simulink model "INCREMENTAL_ENCODER"  (R2019b)
settings: Solver=VariableStepAuto  StartTime=0.0  StopTime=10.0  RelTol=1e-3
undefined symbols (not defined in the file): Ne
libraries: simulink_extras x5, simulink x2
settings Model: Creator=simone  LastModifiedBy=simone
settings ModelReferenceCC: ModelReferenceNumInstancesAllowed=Single

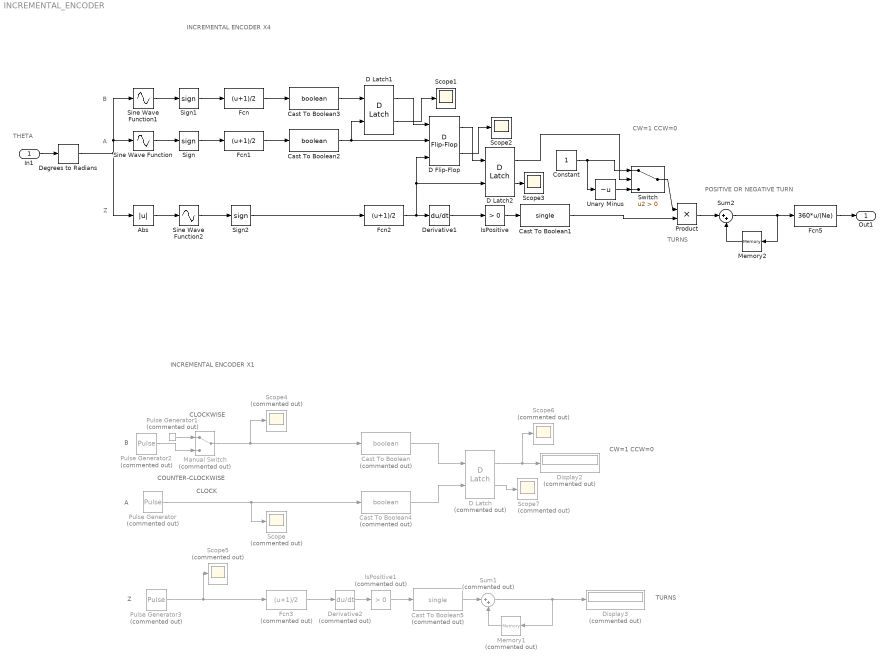
== system INCREMENTAL_ENCODER ==
  note: POSITIVE OR NEGATIVE TURN
  note: THETA
  note: Z
  note: B
  note: CW=1
      | CCW=0
  note: A
  note: INCREMENTAL ENCODER X4
  note: B
  note: TURNS
  note: Z
  note: COUNTER-CLOCKWISE
  note: A
  note: CLOCK
  note: CLOCKWISE
  note: CW=1
      |
      | CCW=0
  note: INCREMENTAL ENCODER X1
  note: TURNS
  In1 : Inport
  Abs : Abs
  Cast To Boolean : DataTypeConversion  Commented=on  OutDataTypeStr=boolean
  Cast To Boolean1 : DataTypeConversion  OutDataTypeStr=single  RndMeth=Zero
  Cast To Boolean2 : DataTypeConversion  OutDataTypeStr=boolean
  Cast To Boolean3 : DataTypeConversion  OutDataTypeStr=boolean  RndMeth=Zero
  Cast To Boolean4 : DataTypeConversion  Commented=on  OutDataTypeStr=boolean
  Cast To Boolean5 : DataTypeConversion  Commented=on  OutDataTypeStr=single  RndMeth=Zero
  Constant : Constant
  D Flip-Flop : simulink_extras/Flip Flops/D Flip-Flop
      settings: SourceProductName=Simulink
  D Latch : simulink_extras/Flip Flops/D Latch  Commented=on
      settings: SourceProductName=Simulink  SourceProductBaseCode=SL
  D Latch1 : simulink_extras/Flip Flops/D Latch
      settings: SourceProductName=Simulink  SourceProductBaseCode=SL
  D Latch2 : simulink_extras/Flip Flops/D Latch
      settings: SourceProductName=Simulink  SourceProductBaseCode=SL
  Degrees to Radians : simulink_extras/Transformations/Degrees to Radians
  Derivative1 : Derivative
  Derivative2 : Derivative  Commented=on
  Display2 : Display  Commented=on
  Display3 : Display  Commented=on
  Fcn : Fcn  Expr=(u+1)/2
  Fcn1 : Fcn  Expr=(u+1)/2
  Fcn2 : Fcn  Expr=(u+1)/2
  Fcn3 : Fcn  Commented=on  Expr=(u+1)/2
  Fcn5 : Fcn  Expr=360*u/(Ne)
  IsPositive : simulink/Logic and Bit Operations/Compare To Zero  relop=>  OutDataTypeStr=boolean
  IsPositive1 : simulink/Logic and Bit Operations/Compare To Zero  Commented=on  relop=>  OutDataTypeStr=boolean
  Manual Switch : ManualSwitch  Commented=on
  Memory1 : Memory  Commented=on  InheritSampleTime=on  LinearizeMemory=on  LinearizeAsDelay=on
  Memory2 : Memory  InitialCondition=-1  InheritSampleTime=on  LinearizeMemory=on  LinearizeAsDelay=on
  Product : Product
  Pulse Generator : DiscretePulseGenerator  Commented=on  PulseType=Time based  Period=1  PulseWidth=50
  Pulse Generator1 : DiscretePulseGenerator  Commented=on  PulseType=Time based  Period=1  PulseWidth=50  PhaseDelay=-0.25
  Pulse Generator2 : DiscretePulseGenerator  Commented=on  PulseType=Time based  Period=1  PulseWidth=50  PhaseDelay=0.25
  Pulse Generator3 : DiscretePulseGenerator  Commented=on  PulseType=Time based  PhaseDelay=2
  Scope{,4..7} (5 alike) : Scope  Commented=on
  Scope1 : Scope
  Scope2 : Scope
  Scope3 : Scope
  Sign : Signum
  Sign1 : Signum
  Sign2 : Signum
  Sine Wave Function : Sin  TimeSource=Use external signal  Frequency=Ne  SampleTime=0
  Sine Wave Function1 : Sin  TimeSource=Use external signal  Frequency=Ne  Phase=-pi/2  SampleTime=0
  Sine Wave Function2 : Sin  TimeSource=Use external signal  Frequency=Ne  SampleTime=0
  Sum1 : Sum  Commented=on  Inputs=|++
  Sum2 : Sum  Inputs=|++
  Switch : Switch  Criteria=u2 > Threshold
  Unary Minus : UnaryMinus
  Out1 : Outport
  wires:
  Degrees to Radians/1 -> Sine Wave Function1/1, Sine Wave Function/1, Abs/1
  Cast To Boolean2/1 -> D Latch1/2, D Flip-Flop/2
  Sign/1 -> Fcn1/1
  Fcn/1 -> Cast To Boolean3/1
  Sign1/1 -> Fcn/1
  D Flip-Flop/1 -> D Latch2/1
  Fcn1/1 -> Cast To Boolean2/1
  Sign2/1 -> Fcn2/1
  IsPositive/1 -> Cast To Boolean1/1
  Sine Wave Function1/1 -> Sign1/1
  Sum2/1 -> Memory2/1, Fcn5/1
  Memory2/1 -> Sum2/2
  Abs/1 -> Sine Wave Function2/1
  Sine Wave Function2/1 -> Sign2/1
  Derivative1/1 -> IsPositive/1
  Fcn2/1 -> D Flip-Flop/3, D Latch2/2, Derivative1/1
  Sine Wave Function/1 -> Sign/1
  In1/1 -> Degrees to Radians/1
  D Latch1/1 -> D Flip-Flop/1
  Cast To Boolean3/1 -> D Latch1/1
  Pulse Generator3/1 -> Scope5/1, Fcn3/1
  Cast To Boolean5/1 -> Sum1/1
  Sum1/1 -> Memory1/1, Display3/1
  Derivative2/1 -> IsPositive1/1
  Cast To Boolean/1 -> D Latch/1
  IsPositive1/1 -> Cast To Boolean5/1
  Pulse Generator2/1 -> Manual Switch/2
  D Latch/1 -> Scope6/1, Display2/1
  Fcn3/1 -> Derivative2/1
  Pulse Generator/1 -> Scope/1, Cast To Boolean4/1
  Pulse Generator1/1 -> Manual Switch/1
  Manual Switch/1 -> Scope4/1, Cast To Boolean/1
  Memory1/1 -> Sum1/2
  Cast To Boolean4/1 -> D Latch/2
  D Latch2/1 -> Switch/2
  Fcn5/1 -> Out1/1
  Product/1 -> Sum2/1
  Switch/1 -> Product/1
  Cast To Boolean1/1 -> Product/2
  Constant/1 -> Unary Minus/1, Switch/1
  Unary Minus/1 -> Switch/3
  D Latch1/2 -> Scope1/1
  D Flip-Flop/2 -> Scope2/1
  D Latch2/2 -> Scope3/1
  D Latch/2 -> Scope7/1
